simulink model "TierPressureMonitoring_git"  (R2020b)
settings: Solver=VariableStepAuto  StartTime=0.0  StopTime=10  RelTol=1e-3
settings Model: Creator=99003728  LastModifiedBy=99003728

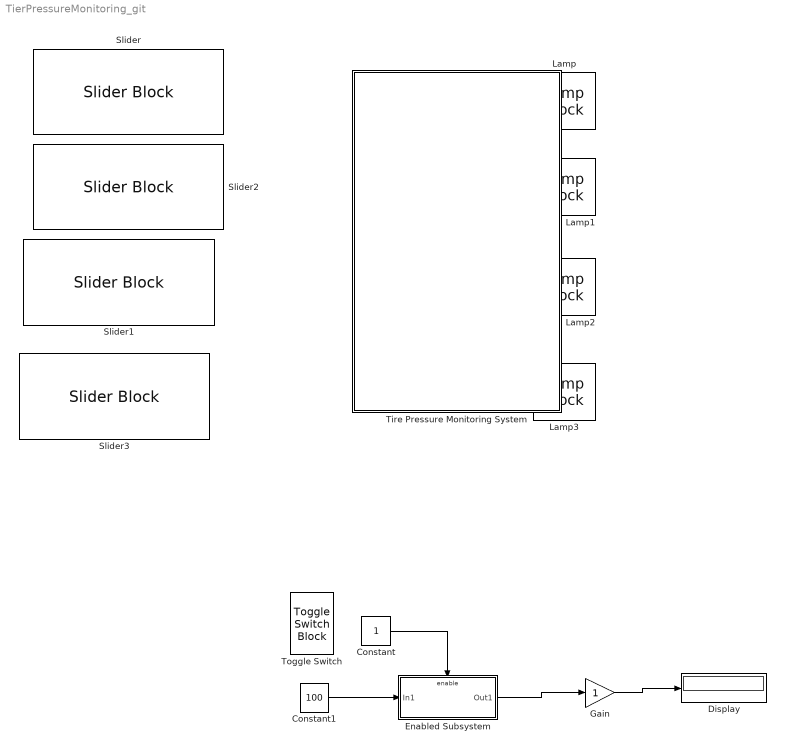
== system TierPressureMonitoring_git ==
  Constant : Constant
  Constant1 : Constant  Value=100
  Display : Display
  Enabled Subsystem : Subsystem  TreatAsAtomicUnit=on
  Gain : Gain
  Lamp{,1..3} (4 alike) : LampBlock
  Slider{,1..3} (4 alike) : SliderBlock
  Tire Pressure Monitoring System : Subsystem
  Toggle Switch : ToggleSwitchBlock
      settings: Values={{'Off', 'On'}, [0 1]}
  wires:
  Constant/1 -> Enabled Subsystem/Enable
  Constant1/1 -> Enabled Subsystem/1(In1)
  Enabled Subsystem/1(Out1) -> Gain/1
  Gain/1 -> Display/1

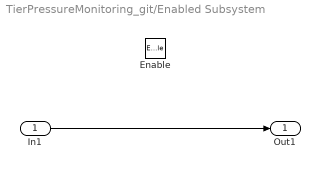
== system TierPressureMonitoring_git/Enabled Subsystem ==
  In1 : Inport
  Enable : EnablePort
  Out1 : Outport
  wires:
  In1/1 -> Out1/1

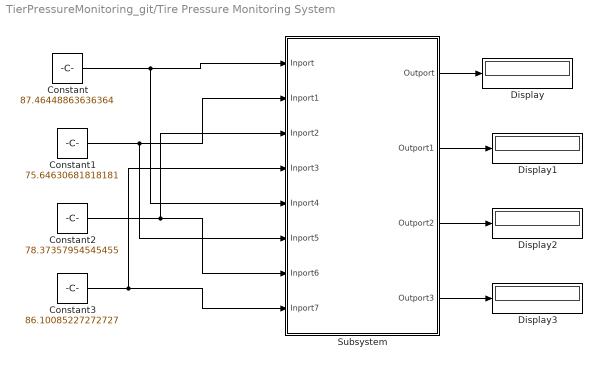
== system TierPressureMonitoring_git/Tire Pressure Monitoring System ==
  Constant : Constant  Value=87.46448863636364
  Constant1 : Constant  Value=75.64630681818181
  Constant2 : Constant  Value=78.37357954545455
  Constant3 : Constant  Value=86.10085227272727
  Display{,1..3} (4 alike) : Display
  Subsystem : Subsystem
  wires:
  Subsystem/2(Outport1) -> Display1/1
  Constant3/1 -> Subsystem/4(Inport3), Subsystem/8(Inport7)
  Subsystem/1(Outport) -> Display/1
  Constant/1 -> Subsystem/5(Inport4), Subsystem/1(Inport)
  Constant2/1 -> Subsystem/3(Inport2), Subsystem/7(Inport6)
  Subsystem/3(Outport2) -> Display2/1
  Constant1/1 -> Subsystem/6(Inport5), Subsystem/2(Inport1)
  Subsystem/4(Outport3) -> Display3/1

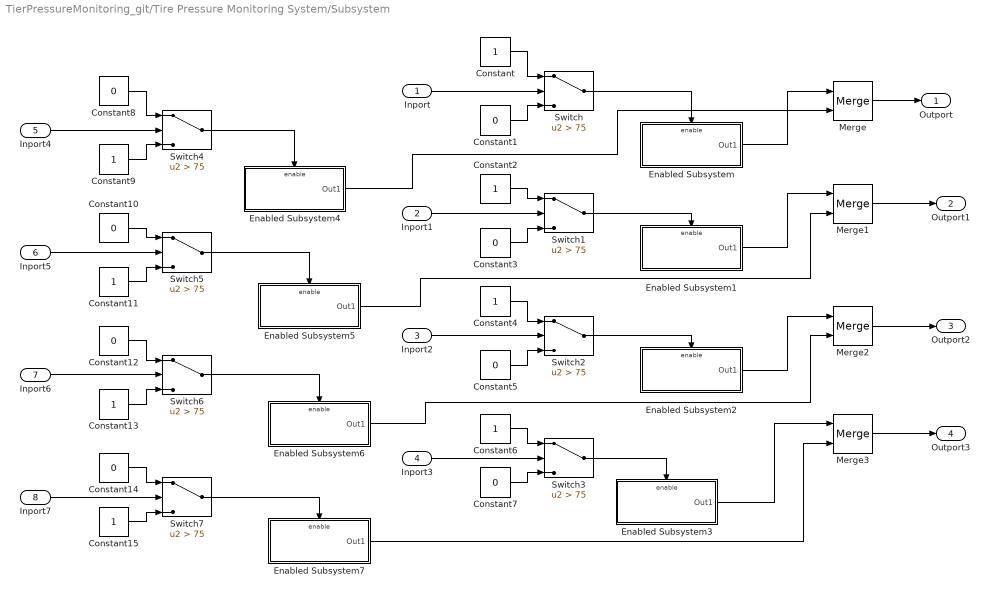
== system TierPressureMonitoring_git/Tire Pressure Monitoring System/Subsystem ==
  Inport : Inport
  Inport1 : Inport  Port=2
  Inport2 : Inport  Port=3
  Inport3 : Inport  Port=4
  Inport4 : Inport  Port=5
  Inport5 : Inport  Port=6
  Inport6 : Inport  Port=7
  Inport7 : Inport  Port=8
  Constant{,2,4,6,9,11,13,15} (8 alike) : Constant
  Constant{1,3,5,7..8,10,12,14} (8 alike) : Constant  Value=0
  Enabled Subsystem : Subsystem  TreatAsAtomicUnit=on
  Enabled Subsystem1 : Subsystem  TreatAsAtomicUnit=on
  Enabled Subsystem2 : Subsystem  TreatAsAtomicUnit=on
  Enabled Subsystem3 : Subsystem  TreatAsAtomicUnit=on
  Enabled Subsystem4 : Subsystem  TreatAsAtomicUnit=on
  Enabled Subsystem5 : Subsystem  TreatAsAtomicUnit=on
  Enabled Subsystem6 : Subsystem  TreatAsAtomicUnit=on
  Enabled Subsystem7 : Subsystem  TreatAsAtomicUnit=on
  Merge{,1..3} (4 alike) : Merge
  Switch{,1..7} (8 alike) : Switch  Criteria=u2 > Threshold  Threshold=75
  Outport : Outport
  Outport1 : Outport  Port=2
  Outport2 : Outport  Port=3
  Outport3 : Outport  Port=4
  wires:
  Constant/1 -> Switch/1
  Inport2/1 -> Switch2/2
  Constant1/1 -> Switch/3
  Constant5/1 -> Switch2/3
  Constant2/1 -> Switch1/1
  Inport/1 -> Switch/2
  Constant7/1 -> Switch3/3
  Constant3/1 -> Switch1/3
  Constant6/1 -> Switch3/1
  Inport1/1 -> Switch1/2
  Inport3/1 -> Switch3/2
  Constant4/1 -> Switch2/1
  Constant14/1 -> Switch7/1
  Constant15/1 -> Switch7/3
  Constant10/1 -> Switch5/1
  Constant11/1 -> Switch5/3
  Constant13/1 -> Switch6/3
  Constant9/1 -> Switch4/3
  Constant8/1 -> Switch4/1
  Inport5/1 -> Switch5/2
  Inport6/1 -> Switch6/2
  Inport4/1 -> Switch4/2
  Constant12/1 -> Switch6/1
  Inport7/1 -> Switch7/2
  Merge/1 -> Outport/1
  Merge1/1 -> Outport1/1
  Merge2/1 -> Outport2/1
  Merge3/1 -> Outport3/1
  Switch3/1 -> Enabled Subsystem3/Enable
  Switch2/1 -> Enabled Subsystem2/Enable
  Switch1/1 -> Enabled Subsystem1/Enable
  Switch/1 -> Enabled Subsystem/Enable
  Switch7/1 -> Enabled Subsystem7/Enable
  Switch6/1 -> Enabled Subsystem6/Enable
  Switch5/1 -> Enabled Subsystem5/Enable
  Switch4/1 -> Enabled Subsystem4/Enable
  Enabled Subsystem/1(Out1) -> Merge/1
  Enabled Subsystem4/1(Out1) -> Merge/2
  Enabled Subsystem1/1(Out1) -> Merge1/1
  Enabled Subsystem5/1(Out1) -> Merge1/2
  Enabled Subsystem2/1(Out1) -> Merge2/1
  Enabled Subsystem6/1(Out1) -> Merge2/2
  Enabled Subsystem3/1(Out1) -> Merge3/1
  Enabled Subsystem7/1(Out1) -> Merge3/2

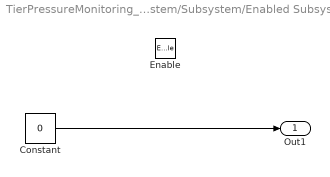
== system TierPressureMonitoring_git/Tire Pressure Monitoring System/Subsystem/Enabled Subsystem ==
  Enable : EnablePort
  Constant : Constant  Value=0
  Out1 : Outport
  wires:
  Constant/1 -> Out1/1

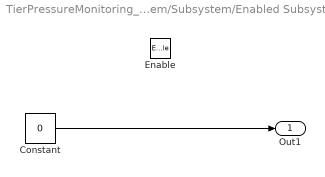
== system TierPressureMonitoring_git/Tire Pressure Monitoring System/Subsystem/Enabled Subsystem1 ==
  Enable : EnablePort
  Constant : Constant  Value=0
  Out1 : Outport
  wires:
  Constant/1 -> Out1/1

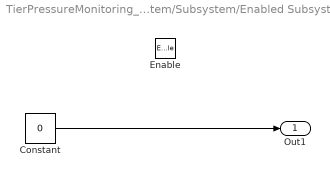
== system TierPressureMonitoring_git/Tire Pressure Monitoring System/Subsystem/Enabled Subsystem2 ==
  Enable : EnablePort
  Constant : Constant  Value=0
  Out1 : Outport
  wires:
  Constant/1 -> Out1/1

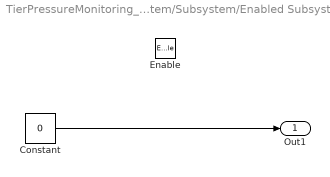
== system TierPressureMonitoring_git/Tire Pressure Monitoring System/Subsystem/Enabled Subsystem3 ==
  Enable : EnablePort
  Constant : Constant  Value=0
  Out1 : Outport
  wires:
  Constant/1 -> Out1/1

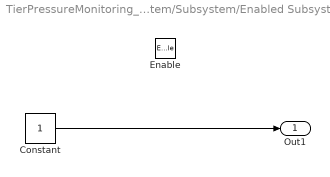
== system TierPressureMonitoring_git/Tire Pressure Monitoring System/Subsystem/Enabled Subsystem4 ==
  Enable : EnablePort
  Constant : Constant
  Out1 : Outport
  wires:
  Constant/1 -> Out1/1

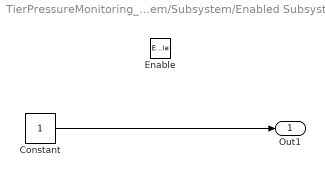
== system TierPressureMonitoring_git/Tire Pressure Monitoring System/Subsystem/Enabled Subsystem5 ==
  Enable : EnablePort
  Constant : Constant
  Out1 : Outport
  wires:
  Constant/1 -> Out1/1

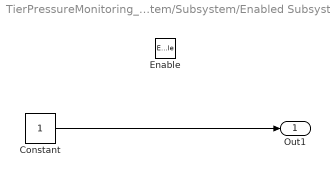
== system TierPressureMonitoring_git/Tire Pressure Monitoring System/Subsystem/Enabled Subsystem6 ==
  Enable : EnablePort
  Constant : Constant
  Out1 : Outport
  wires:
  Constant/1 -> Out1/1

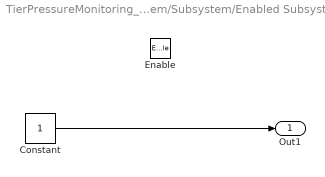
== system TierPressureMonitoring_git/Tire Pressure Monitoring System/Subsystem/Enabled Subsystem7 ==
  Enable : EnablePort
  Constant : Constant
  Out1 : Outport
  wires:
  Constant/1 -> Out1/1
